simulink model "two_virtual_wheel_analog"  (R2020a)
settings: Solver=ode3  StartTime=0.0  StopTime=tfinal  FixedStep=Deltat  RelTol=1e-3  EnableMultiTasking=on
values from neighbouring files (symbols this model uses):
  Jw1 = .5*1.5/4    (= 0.1875)    [two_virtual_wheel_params.m]
  Jw2 = 0.0721    [two_virtual_wheel_params.m]
  k1 = .5*15    (= 7.5)    [two_virtual_wheel_params.m]
  k2 = 3.75    [two_virtual_wheel_params.m]
  step_time = 1    [two_virtual_wheel_params.m]
  Theta_z_0 = 45    [two_virtual_wheel_params.m]
settings Model: ExtModeTrigMode=oneshot  ExtModeArmWhenConnect=off  Creator=jfr  LastModifiedBy=jfr
settings DataIOCC: SaveFormat=Array  SignalLoggingSaveFormat=ModelDataLogs  ReturnWorkspaceOutputs=off
settings OptimizationCC: BooleanDataType=off  InitFltsAndDblsToZero=on  LifeSpan=inf
settings DebuggingCC: SaveWithParameterizedLinksMsg=none  UnderspecifiedInitializationDetection=Classic  MergeDetectMultiDrivingBlocksExec=none  SignalResolutionControl=TryResolveAllWithWarning  MultiTaskDSMMsg=warning  MultiTaskCondExecSysMsg=none  FcnCallInpInsideContextMsg=warning  AllowSymbolicDim=off  SFUnexpectedBacktrackingDiag=warning  SFNoUnconditionalDefaultTransitionDiag=warning  SFExecutionAtInitializationDiag=none  ArithmeticOperatorsInVariantConditions=warning
settings HardwareCC: ProdBitPerPointer=32  ProdBitPerSizeT=32  ProdBitPerPtrDiffT=32  ProdLargestAtomicFloat=None  ProdIntDivRoundTo=Undefined  ProdEndianess=Unspecified  ProdWordSize=32  ProdHWDeviceType=32-bit Generic  TargetUnknown=on
settings ModelReferenceCC: PropagateSignalLabelsOutOfModel=off
settings SFSimCC: SimUseLocalCustomCode=off  CustomCodeUndefinedFunction=UseInterfaceOnly
settings RTWCC: RTWUseLocalCustomCode=off
settings CodeAppCC: StateflowObjectComments=on
settings GRTTargetCC: TargetFcnLib=ansi_tfl_tmw.mat  TargetLangStandard=C89/C90 (ANSI)  CombineOutputUpdateFcns=off  GRTInterface=on
settings ConfigComp: CovMetricSettings=dw  CovHtmlReporting=on  CovSaveCumulativeToWorkspaceVar=on  CovSaveSingleToWorkspaceVar=on  CovExternalEMLEnable=off

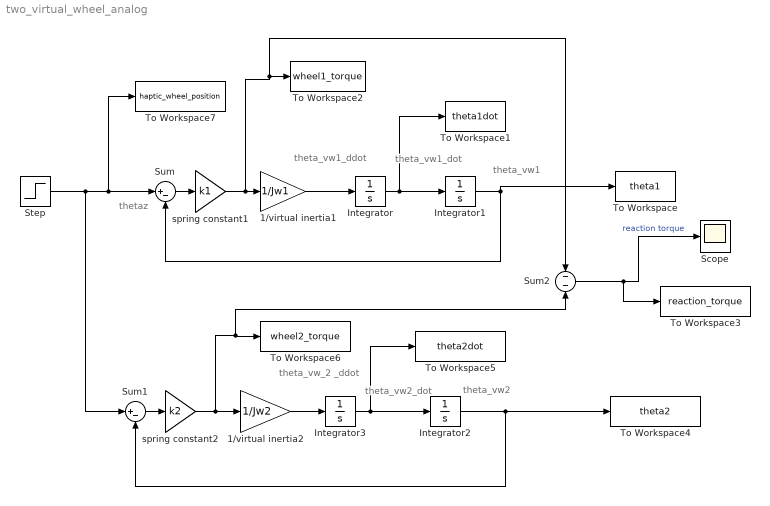
== system two_virtual_wheel_analog ==
  note: theta_vw1
  note: theta_vw1_dot
  note: theta_vw1_ddot
  note: thetaz
  note: theta_vw2
  note: theta_vw2_dot
  note: theta_vw_2
      | _ddot
  1/virtual inertia1 : Gain  Gain=1/Jw1  SaturateOnIntegerOverflow=on  OutDataTypeStr=Inherit: Same as input  ParamDataTypeStr=Inherit: Same as input
  1/virtual inertia2 : Gain  Gain=1/Jw2  SaturateOnIntegerOverflow=on  OutDataTypeStr=Inherit: Same as input  ParamDataTypeStr=Inherit: Same as input
  Integrator{,1..3} (4 alike) : Integrator
  Scope : Scope
  Step : Step  Time=step_time  After=Theta_z_0  SampleTime=0
  Sum : Sum  Inputs=|+-  InputSameDT=on  SaturateOnIntegerOverflow=on  OutDataTypeStr=Inherit: Same as first input
  Sum1 : Sum  Inputs=|+-  InputSameDT=on  SaturateOnIntegerOverflow=on  OutDataTypeStr=Inherit: Same as first input
  Sum2 : Sum  Inputs=-|-  InputSameDT=on  SaturateOnIntegerOverflow=on  OutDataTypeStr=Inherit: Same as first input
  To Workspace : ToWorkspace  VariableName=theta1  SaveFormat=Timeseries  SampleTime=-1
  To Workspace1 : ToWorkspace  VariableName=theta1dot  SaveFormat=Timeseries  SampleTime=-1
  To Workspace2 : ToWorkspace  VariableName=wheel1_torque  SaveFormat=Timeseries  SampleTime=-1
  To Workspace3 : ToWorkspace  VariableName=reaction_torque  SaveFormat=Timeseries  SampleTime=-1
  To Workspace4 : ToWorkspace  VariableName=theta2  SaveFormat=Timeseries  SampleTime=-1
  To Workspace5 : ToWorkspace  VariableName=theta2dot  SaveFormat=Timeseries  SampleTime=-1
  To Workspace6 : ToWorkspace  VariableName=wheel2_torque  SaveFormat=Timeseries  SampleTime=-1
  To Workspace7 : ToWorkspace  VariableName=haptic_wheel_position  SaveFormat=Timeseries  SampleTime=-1
  spring constant1 : Gain  Gain=k1  SaturateOnIntegerOverflow=on  OutDataTypeStr=Inherit: Same as input  ParamDataTypeStr=Inherit: Same as input
  spring constant2 : Gain  Gain=k2  SaturateOnIntegerOverflow=on  OutDataTypeStr=Inherit: Same as input  ParamDataTypeStr=Inherit: Same as input
  wires:
  Integrator1/1 -> To Workspace/1, Sum/2
  Sum/1 -> spring constant1/1
  Step/1 -> To Workspace7/1, Sum/1, Sum1/1
  1/virtual inertia1/1 -> Integrator/1
  Integrator/1 -> Integrator1/1, To Workspace1/1
  Integrator2/1 -> To Workspace4/1, Sum1/2
  Sum1/1 -> spring constant2/1
  1/virtual inertia2/1 -> Integrator3/1
  Integrator3/1 -> To Workspace5/1, Integrator2/1
  Sum2/1 -> To Workspace3/1, Scope/1  "reaction torque"
  spring constant1/1 -> 1/virtual inertia1/1, To Workspace2/1, Sum2/1
  spring constant2/1 -> 1/virtual inertia2/1, To Workspace6/1, Sum2/2
